simulink model "newfour"  (R2021a)
settings: Solver=VariableStepAuto  StartTime=0.0  StopTime=688000  RelTol=1e-3
values from neighbouring files (symbols this model uses):
  Ts = 0.5    [Distillation_Column_model_identification.m]    (also in Distillation_Column_model_variance.m; fourvary.m = 8)
libraries: cstblocks x2, dspsrcs4 x1
settings Model: Creator=dell  LastModifiedBy=dell
settings DataIOCC: LoadExternalInput=on

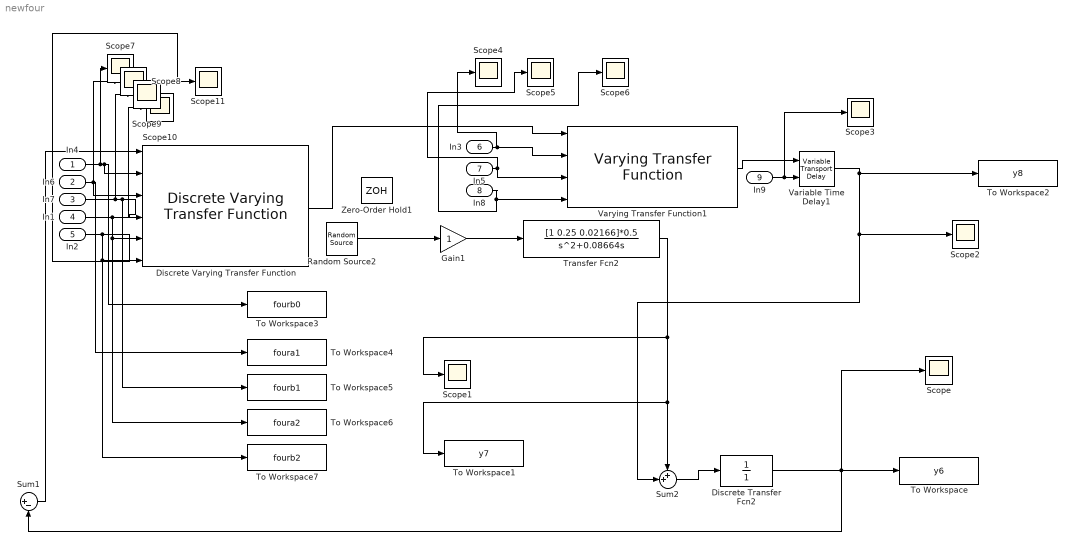
== system newfour ==
  In4 : Inport
  In6 : Inport  Port=2
  In7 : Inport  Port=3
  In1 : Inport  Port=4
  In2 : Inport  Port=5
  In3 : Inport  Port=6
  In5 : Inport  Port=7
  In8 : Inport  Port=8
  In9 : Inport  Port=9
  Discrete Transfer Fcn2 : DiscreteTransferFcn  Denominator=[1]  SampleTime=Ts
      mask Display: disp('sampler')
  Discrete Varying Transfer Function : cstblocks/Linear Parameter Varying/Discrete Varying Transfer Function  N=2  Ts=Ts
      settings: SourceProductBaseCode=CT
  Gain1 : Gain
  Random Source2 : dspsrcs4/Random Source  SrcType=Gaussian  NormMethod=Ziggurat  CltLength=12  MinVal=-1  MaxVal=1  MeanVal=0  VarVal=1  RepMode=Specify seed  rawSeed=seed  IsInherit=off  SampMode=Continuous  SampTime=1  SampFrame=1  DataType=Double  OutComplex=Real  OutputFrames=off
  Scope{,1..11} (12 alike) : Scope
  Sum1 : Sum  Inputs=|+-
  Sum2 : Sum  Inputs=++|
  To Workspace : ToWorkspace  VariableName=y6  SampleTime=Ts
  To Workspace1 : ToWorkspace  VariableName=y7  SampleTime=Ts
  To Workspace2 : ToWorkspace  VariableName=y8  SampleTime=Ts
  To Workspace3 : ToWorkspace  VariableName=fourb0  SampleTime=Ts
  To Workspace4 : ToWorkspace  VariableName=foura1  SampleTime=Ts
  To Workspace5 : ToWorkspace  VariableName=fourb1  SampleTime=Ts
  To Workspace6 : ToWorkspace  VariableName=foura2  SampleTime=Ts
  To Workspace7 : ToWorkspace  VariableName=fourb2  SampleTime=Ts
  Transfer Fcn2 : TransferFcn  Numerator=[1 0.25 0.02166]*0.5  Denominator=[1 0.08664 0]
  Variable Time Delay1 : VariableTransportDelay  MaximumDelay=200
  Varying Transfer Function1 : cstblocks/Linear Parameter Varying/Varying Transfer Function  N=1
  Zero-Order Hold1 : ZeroOrderHold  SampleTime=Ts
  wires:
  Variable Time Delay1/1 -> To Workspace2/1, Scope2/1, Sum2/2
  In9/1 -> Scope3/1, Variable Time Delay1/2
  Sum1/1 -> Discrete Varying Transfer Function/1
  In8/1 -> Scope6/1, Varying Transfer Function1/4
  In6/1 -> Discrete Varying Transfer Function/3, To Workspace4/1, Scope8/1
  In1/1 -> Discrete Varying Transfer Function/5, To Workspace6/1, Scope10/1
  Sum2/1 -> Discrete Transfer Fcn2/1
  Transfer Fcn2/1 -> Scope1/1, To Workspace1/1, Sum2/1
  In3/1 -> Scope4/1, Varying Transfer Function1/2
  Discrete Transfer Fcn2/1 -> Scope/1, Sum1/2, To Workspace/1
  Random Source2/1 -> Gain1/1
  In4/1 -> Scope7/1, Discrete Varying Transfer Function/2, To Workspace3/1
  In7/1 -> Discrete Varying Transfer Function/4, To Workspace5/1, Scope9/1
  In5/1 -> Scope5/1, Varying Transfer Function1/3
  In2/1 -> Discrete Varying Transfer Function/6, To Workspace7/1, Scope11/1
  Gain1/1 -> Transfer Fcn2/1
  Varying Transfer Function1/1 -> Variable Time Delay1/1
  Discrete Varying Transfer Function/1 -> Varying Transfer Function1/1
